simulink model "decoder"  (R2022a)
settings: Solver=VariableStepAuto  StartTime=0.0  StopTime=10.0  RelTol=1e-3
settings Model: Creator=cuomo  LastModifiedBy=cuomo

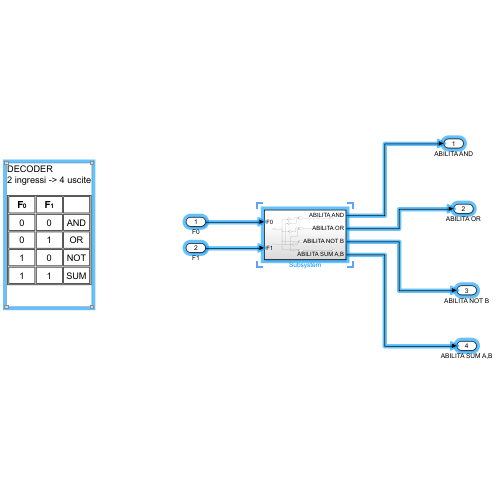
[thumbnail: Simulink's stored preview of the top-level diagram]
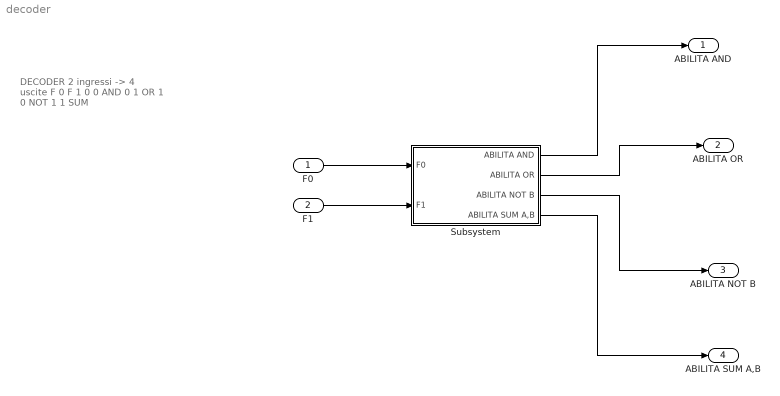
== system decoder ==
  note: DECODER
      | 2 ingressi -> 4 uscite
      |
      | F 0
      | F 1
      |
      | 0
      | 0
      | AND
      |
      | 0
      | 1
      | OR
      |
      | 1
      | 0
      | NOT
      |
      | 1
      | 1
      | SUM
  F0 : Inport
  F1 : Inport  Port=2
  Subsystem : Subsystem
  ABILITA AND : Outport
  ABILITA OR : Outport  Port=2
  ABILITA NOT B : Outport  Port=3
  ABILITA SUM A,B : Outport  Port=4
  wires:
  Subsystem/3(ABILITA NOT B) -> ABILITA NOT B/1
  F1/1 -> Subsystem/2(F1)
  F0/1 -> Subsystem/1(F0)
  Subsystem/1(ABILITA AND) -> ABILITA AND/1
  Subsystem/4(ABILITA SUM A,B) -> ABILITA SUM A,B/1
  Subsystem/2(ABILITA OR) -> ABILITA OR/1

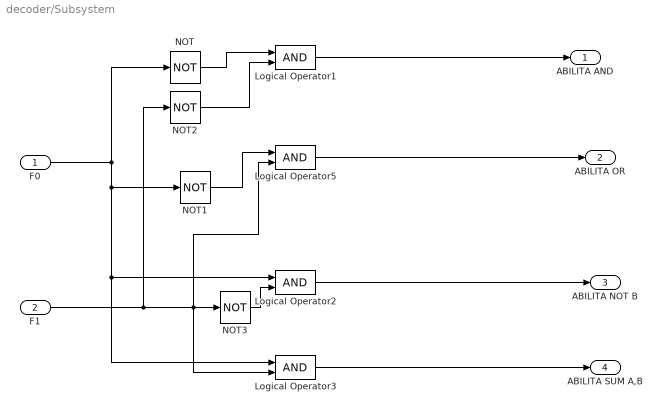
== system decoder/Subsystem ==
  F0 : Inport
  F1 : Inport  Port=2
  Logical Operator{1..3,5} (4 alike) : Logic  IconShape=distinctive  AllPortsSameDT=off  OutDataTypeStr=boolean
  NOT{,1..3} (4 alike) : Logic  Operator=NOT  IconShape=distinctive  AllPortsSameDT=off  OutDataTypeStr=boolean
  ABILITA AND : Outport
  ABILITA OR : Outport  Port=2
  ABILITA NOT B : Outport  Port=3
  ABILITA SUM A,B : Outport  Port=4
  wires:
  NOT2/1 -> Logical Operator1/2
  F0/1 -> Logical Operator3/1, Logical Operator2/1, NOT1/1, NOT/1
  F1/1 -> NOT2/1, Logical Operator3/2, Logical Operator5/2, NOT3/1
  Logical Operator5/1 -> ABILITA OR/1
  Logical Operator2/1 -> ABILITA NOT B/1
  NOT3/1 -> Logical Operator2/2
  Logical Operator3/1 -> ABILITA SUM A,B/1
  NOT1/1 -> Logical Operator5/1
  Logical Operator1/1 -> ABILITA AND/1
  NOT/1 -> Logical Operator1/1
